simulink model "lab_2_2"  (R2020b)
settings: Solver=ode45  StartTime=0.0  StopTime=30  RelTol=1e-8
settings Model: Creator=whitehole  LastModifiedBy=whitehole

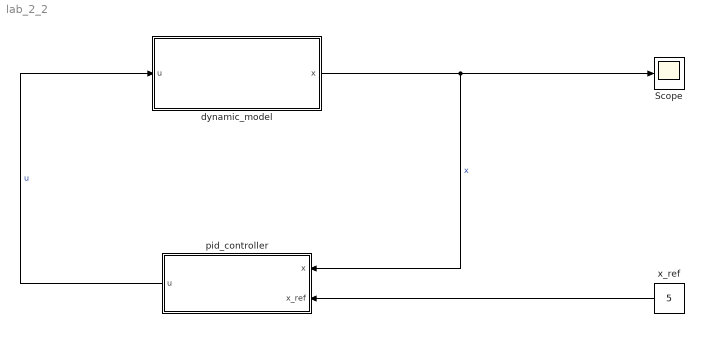
== system lab_2_2 ==
  Scope : Scope
  dynamic_model : Subsystem
  pid_controller : Subsystem
  x_ref : Constant  Value=5
  wires:
  dynamic_model/1(x) -> pid_controller/1(x), Scope/1  "x"
  pid_controller/1(u) -> dynamic_model/1(u)  "u"
  x_ref/1 -> pid_controller/2(x_ref)

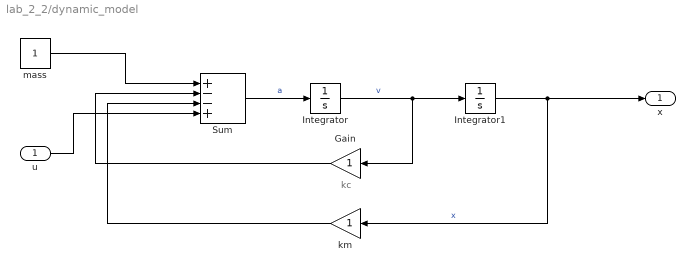
== system lab_2_2/dynamic_model ==
  note: kc
  u : Inport
  Gain : Gain
  Integrator : Integrator
  Integrator1 : Integrator
  Sum : Sum  Inputs=+|-|-|+
  km : Gain
  mass : Constant
  x : Outport
  wires:
  mass/1 -> Sum/1
  u/1 -> Sum/4
  Sum/1 -> Integrator/1  "a"
  Integrator1/1 -> x/1, km/1  "x"
  km/1 -> Sum/3
  Gain/1 -> Sum/2
  Integrator/1 -> Gain/1, Integrator1/1  "v"

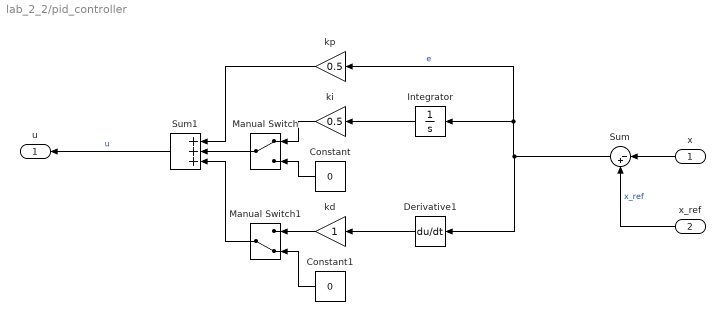
== system lab_2_2/pid_controller ==
  x : Inport
  x_ref : Inport  Port=2
  Constant : Constant  Value=0
  Constant1 : Constant  Value=0
  Derivative1 : Derivative
  Integrator : Integrator
  Manual Switch : ManualSwitch
  Manual Switch1 : ManualSwitch  CurrentSetting=0
  Sum : Sum  Inputs=|-+
  Sum1 : Sum  Inputs=+++
  kd : Gain
  ki : Gain  Gain=0.5
  kp : Gain  Gain=0.5
  u : Outport
  wires:
  kp/1 -> Sum1/1
  Sum1/1 -> u/1  "u"
  x_ref/1 -> Sum/2  "x_ref"
  x/1 -> Sum/1
  Sum/1 -> kp/1, Integrator/1, Derivative1/1  "e"
  Integrator/1 -> ki/1
  ki/1 -> Manual Switch/1
  Derivative1/1 -> kd/1
  kd/1 -> Manual Switch1/1
  Manual Switch/1 -> Sum1/2
  Constant/1 -> Manual Switch/2
  Manual Switch1/1 -> Sum1/3
  Constant1/1 -> Manual Switch1/2
